simulink model "ereignis_zustand_umwandlung"  (R2015b)
settings: Solver=FixedStepAuto  StartTime=0.0  StopTime=10.0  RelTol=1e-3
libraries: simulink x1
settings Model: Creator=scco1019  LastModifiedBy=scco1019

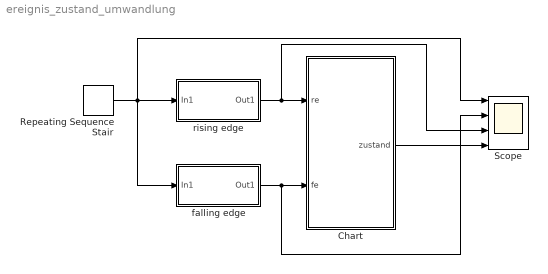
== system ereignis_zustand_umwandlung ==
  Chart : Stateflow chart  TreatAsAtomicUnit=on
  Repeating Sequence Stair : simulink/Sources/Repeating Sequence Stair  OutValues=[1 0 1 1 1 1 0 1 0 0 1 0 1].'  tsamp=-1  OutMin=[]  OutMax=[]  OutDataTypeStr=double  OutputDataTypeScalingMode=double  OutDataType=fixdt(0,8)  ConRadixGroup=Best Precision: Vector-wise  OutScaling=2^-12
  Scope : Scope  NumInputPorts=4
  falling edge : Subsystem
  rising edge : Subsystem
  wires:
  Repeating Sequence Stair/1 -> Scope/1, falling edge/1(In1), rising edge/1(In1)
  rising edge/1(Out1) -> Scope/3, Chart/1(re)
  falling edge/1(Out1) -> Scope/2, Chart/2(fe)
  Chart/1(zustand) -> Scope/4

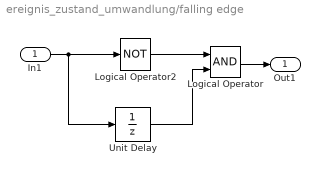
== system ereignis_zustand_umwandlung/falling edge ==
  In1 : Inport
  Logical Operator : Logic  AllPortsSameDT=off  OutDataTypeStr=boolean
  Logical Operator2 : Logic  Operator=NOT  AllPortsSameDT=off  OutDataTypeStr=boolean
  Unit Delay : UnitDelay  SampleTime=-1
  Out1 : Outport
  wires:
  Unit Delay/1 -> Logical Operator/2
  Logical Operator/1 -> Out1/1
  In1/1 -> Unit Delay/1, Logical Operator2/1
  Logical Operator2/1 -> Logical Operator/1

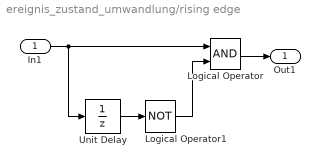
== system ereignis_zustand_umwandlung/rising edge ==
  In1 : Inport
  Logical Operator : Logic  AllPortsSameDT=off  OutDataTypeStr=boolean
  Logical Operator1 : Logic  Operator=NOT  AllPortsSameDT=off  OutDataTypeStr=boolean
  Unit Delay : UnitDelay  SampleTime=-1
  Out1 : Outport
  wires:
  In1/1 -> Logical Operator/1, Unit Delay/1
  Logical Operator/1 -> Out1/1
  Unit Delay/1 -> Logical Operator1/1
  Logical Operator1/1 -> Logical Operator/2

== stateflow chart ereignis_zustand_umwandlung/Chart ==
  state Zustand_0/
    entry: zustand=0;
  state Zustand_1/
    entry: zustand=1;
  (default) -> Zustand_0
  Zustand_0 -> Zustand_0 [order 2]
  Zustand_1 -> Zustand_0 [order 1] : [fe==1]
  Zustand_0 -> Zustand_1 [order 1] : [re==1]
  Zustand_1 -> Zustand_1 [order 2]
  data: zustand output; re input; fe input
